simulink model "system_model_optim"  (R2021a)
settings: Solver=VariableStepAuto  StartTime=0.0  StopTime=SimEndTime  RelTol=1e-3
undefined symbols (not defined in the file): ctrl_start_time, Iout_ref, TimeStep
libraries: checkpacklib x1, simulink x1, SignalEditorBlockLib x1
settings Model: DataDictionary=system_data.sldd  Creator=tshintai  LastModifiedBy=tshintai
settings SolverCC: AlgebraicLoopSolver=TrustRegion
settings DebuggingCC: SFMachineParentedDataDiag=warning

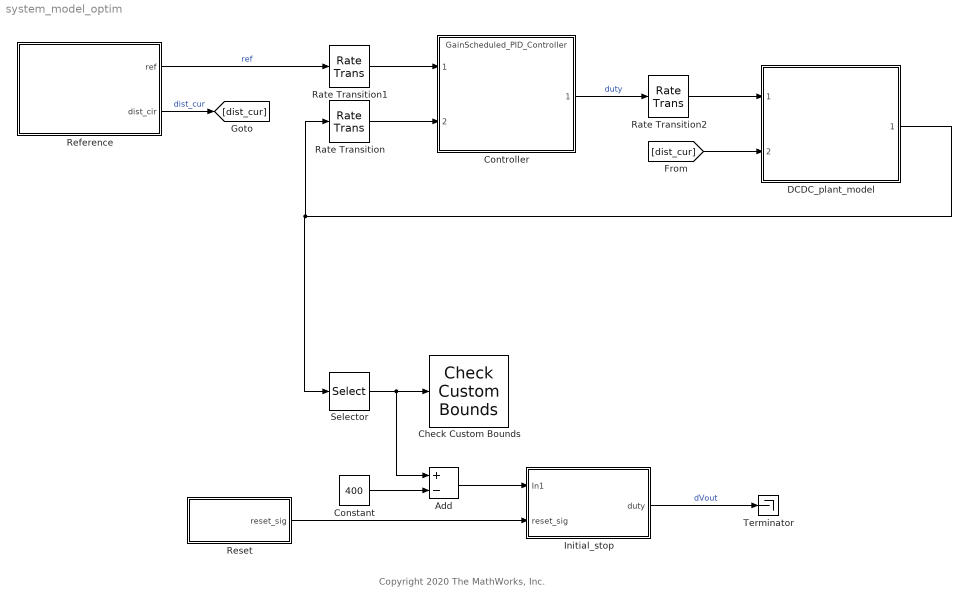
== system system_model_optim ==
  note: Copyright 2020 The MathWorks, Inc.
  Add : Sum  Inputs=+-
  Check Custom Bounds : checkpacklib/Check Custom Bounds  InstantiateOnLoad=on  enabled=off  stopWhenAssertionFail=off  export=off  ViewDlgPos=[1085 264 510 390]  OpenViewOnLoad=off  LaunchViewOnOpen=off  TimeUnits=seconds  EnableUpperBound=on  UpperBoundTimes=[0 0.8]  UpperBoundAmplitudes=[420 420];  EnableLowerBound=on  LowerBoundTimes=[0 0.01; 0.01, 0.8]  LowerBoundAmplitudes=[0, 0; 380 380]
      settings: SourceProductBaseCode=CT,ID,MT,SO
  Constant : Constant  Value=400
  Controller : ModelReference  ModelNameDialog=GainScheduled_PID_Controller  SimulationMode=Normal  ModelReferenceVersion=2.1
  DCDC_plant_model : Subsystem  ReferencedSubsystem=DCDC_plant_model
  Initial_stop : Subsystem
  Rate Transition : RateTransition  OutPortSampleTime=TimeStep
  Rate Transition1 : RateTransition  OutPortSampleTime=TimeStep
  Rate Transition2 : RateTransition
  Reference : Subsystem
  Reset : Subsystem
  Selector : Selector  InputPortWidth=3  IndexOptions=Index vector (dialog)  Indices=[2]  OutputSizes=1
  Terminator : Terminator
  wires:
  Controller/1 -> Rate Transition2/1  "duty"
  DCDC_plant_model/1 -> Selector/1, Rate Transition/1
  Reference/1(ref) -> Rate Transition1/1  "ref"
  Rate Transition/1 -> Controller/2
  Rate Transition1/1 -> Controller/1
  Rate Transition2/1 -> DCDC_plant_model/1
  Reference/2(dist_cir) -> [dist_cur]  "dist_cur"
  [dist_cur] -> DCDC_plant_model/2
  Selector/1 -> Add/1, Check Custom Bounds/1
  Initial_stop/1(duty) -> Terminator/1  "dVout"
  Reset/1(reset_sig) -> Initial_stop/2(reset_sig)
  Constant/1 -> Add/2
  Add/1 -> Initial_stop/1(In1)

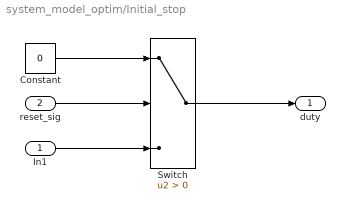
== system system_model_optim/Initial_stop ==
  In1 : Inport
  reset_sig : Inport  Port=2
  Constant : Constant  Value=0
  Switch : Switch  Criteria=u2 > Threshold
  duty : Outport
  wires:
  reset_sig/1 -> Switch/2
  Switch/1 -> duty/1
  Constant/1 -> Switch/1
  In1/1 -> Switch/3

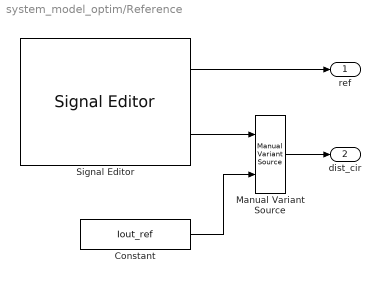
== system system_model_optim/Reference ==
  Constant : Constant  Value=Iout_ref
  Manual Variant Source : simulink/Signal Routing/Manual Variant Source  NumChoices=2  LabelModeActiveChoice=V_1
  Signal Editor : SignalEditorBlockLib/Signal Editor  FileName=ref_signal.mat  ActiveScenario=Step_current_work  ActiveSignal=Vref  IsBus=off  OutputBusObjectStr=Bus: BusObject  SampleTime=0  ZeroCross=off  OutputAfterFinalValue=Holding final value  Unit=inherit  PreserveSignalName=on
  ref : Outport
  dist_cir : Outport  Port=2
  wires:
  Signal Editor/1 -> ref/1
  Signal Editor/2 -> Manual Variant Source/1
  Manual Variant Source/1 -> dist_cir/1
  Constant/1 -> Manual Variant Source/2

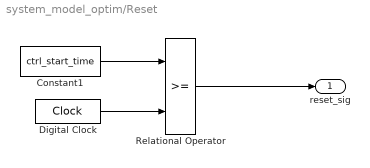
== system system_model_optim/Reset ==
  Constant1 : Constant  Value=ctrl_start_time
  Digital Clock : DigitalClock  SampleTime=TimeStep
  Relational Operator : RelationalOperator  OutDataTypeStr=boolean  RndMeth=Simplest
  reset_sig : Outport
  wires:
  Relational Operator/1 -> reset_sig/1
  Digital Clock/1 -> Relational Operator/2
  Constant1/1 -> Relational Operator/1
